simulink model "sampleModel1801"  (R2022a)
settings: Solver=FixedStepAuto  StartTime=0.0  StopTime=10.0  RelTol=1e-3
undefined symbols (not defined in the file): DiscIntNeverNeededParam, Newton, Raphson
libraries: simulink x66, slpidlib x17
(part 1 of 3)
settings Model: SimulationMode=software-in-the-loop (sil)  Creator=lenovo  LastModifiedBy=TSMC
settings DataIOCC: InspectSignalLogs=on  SignalLoggingName=logsOut
settings OptimizationCC: DefaultParameterBehavior=Inlined  EnhancedBackFolding=on  PassReuseOutputArgsAs=Individual arguments  ZeroExternalMemoryAtStartup=off  ZeroInternalMemoryAtStartup=off  OptimizeBlockOrder=speed  DifferentSizesBufferReuse=on  OptimizationCustomize=off  EfficientTunableParamExpr=on
settings DebuggingCC: ParameterTunabilityLossMsg=error  UnconnectedInputMsg=warning  UnconnectedOutputMsg=warning  UnconnectedLineMsg=warning
settings ModelReferenceCC: UpdateModelReferenceTargets=Force
settings SFSimCC: MATLABDynamicMemAlloc=off
settings RTWCC: SystemTargetFile=ert.tlc  TemplateMakefile=ert_default_tmf  GenerateReport=on  IncludeHyperlinkInReport=on  GenerateTraceInfo=on  DLArmComputeVersion=19.05
settings CodeAppCC: ForceParamTrailComments=on  IgnoreCustomStorageClasses=off  OperatorAnnotations=on  SimulinkDataObjDesc=on  SFDataObjDesc=on  InsertBlockDesc=on
settings ERTTargetCC: TargetLangStandard=C99 (ISO)  GenerateSampleERTMain=on  SupportContinuousTime=on  InlinedParameterPlacement=NonHierarchical  ERTCustomFileTemplate=example_file_process.tlc

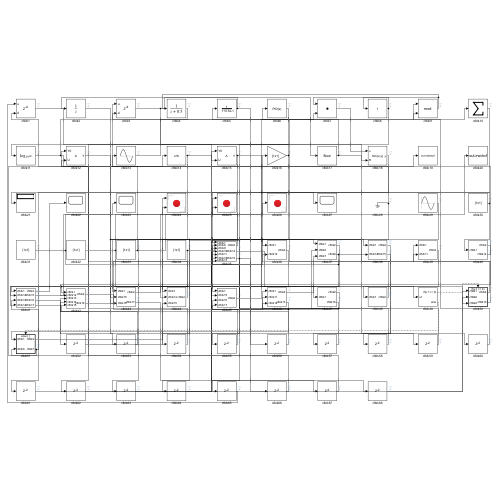
[thumbnail: Simulink's stored preview of the top-level diagram]
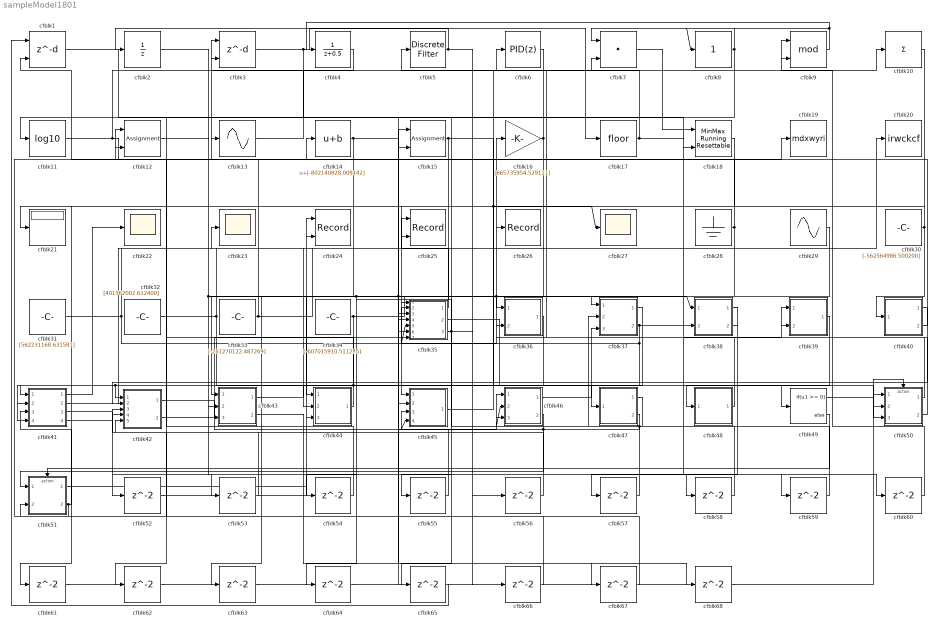
== system sampleModel1801 ==
  cfblk1 : Delay  DelayLengthSource=Input port  SampleTime=1
      settings: InputPortMap=u0,p1
  cfblk10 : Sum  Inputs=+
  cfblk11 : Math  Operator=log10
  cfblk12 : Assignment  DiagnosticForDimensions=Warning  IndexOptions=Index vector (dialog)  Indices=1  OutputSizes=1
  cfblk13 : Sin  TimeSource=Use external signal  SampleTime=0
  cfblk14 : Bias  Bias=[-802140828.008142]  SaturateOnIntegerOverflow=off
  cfblk15 : Assignment  DiagnosticForDimensions=Warning  IndexOptions=Index vector (dialog)  Indices=1  OutputSizes=1
  cfblk16 : Gain  Gain=[665735954.529111]
  cfblk17 : Rounding
  cfblk18 : simulink/Math Operations/MinMax Running Resettable  Function=min  vinit=0.0
  cfblk19 : ToWorkspace  VariableName=mdxwyri  SaveFormat=Timeseries  SampleTime=-1
  cfblk2 : UnitDelay  HasFrameUpgradeWarning=on
  cfblk20 : ToWorkspace  VariableName=irwckcf  SaveFormat=Timeseries  SampleTime=-1
  cfblk21 : Display
  cfblk22 : Scope
  cfblk23 : Scope
  cfblk24 : Record  FileSettingsInternal="{\"entries\":[{\"content\":{\"excelSettings\":{\"content\":{},\"type\":\"Streamout.ExcelSettings\"}},\"type\":\"Streamout.FileSettingStorage\",\"uuid\":\"da407134-930a-4060-90fa-d972cd5884a4\"}],\"packageUris\":[\"http://schema.mathworks.com/mf0/streamout_blocks/R2020a\"],\"version\":\"1.0\"}"  Layout=[1 1]  SignalsInternal="{\"entries\":[{\"content\":{\"signals\":[]},\"type\":\"RecordBlkView.InputSignals\",\"uuid\":\"b8d77bba-2430-47da-b420-9572af3fcd64\"}],\"packageUris\":[\"http://schema.mathworks.com/mf0/streamout_blocks/R2020a\"],\"version\":\"1.0\"}"  VisualizationBindings="{\"xyplotplugin\":{\"info\":[{\"series\":[],\"subplotID\":1}]}}"  CompatibilityTag=XY  st=-1
  cfblk25 : Record  FileSettingsInternal="{\"entries\":[{\"content\":{\"excelSettings\":{\"content\":{},\"type\":\"Streamout.ExcelSettings\"}},\"type\":\"Streamout.FileSettingStorage\",\"uuid\":\"0478fcfe-5d0e-44ee-9fcd-b61e8d59bef5\"}],\"packageUris\":[\"http://schema.mathworks.com/mf0/streamout_blocks/R2020a\"],\"version\":\"1.0\"}"  Layout=[1 1]  SignalsInternal="{\"entries\":[{\"content\":{\"signals\":[]},\"type\":\"RecordBlkView.InputSignals\",\"uuid\":\"ba91bab0-cdaa-4586-8070-7859b16663df\"}],\"packageUris\":[\"http://schema.mathworks.com/mf0/streamout_blocks/R2020a\"],\"version\":\"1.0\"}"  VisualizationBindings="{\"xyplotplugin\":{\"info\":[{\"series\":[],\"subplotID\":1}]}}"  CompatibilityTag=XY  st=-1
  cfblk26 : Record  FileSettingsInternal="{\"entries\":[{\"content\":{\"excelSettings\":{\"content\":{},\"type\":\"Streamout.ExcelSettings\"}},\"type\":\"Streamout.FileSettingStorage\",\"uuid\":\"70eb35dc-156c-423f-ab29-1b62ce158527\"}],\"packageUris\":[\"http://schema.mathworks.com/mf0/streamout_blocks/R2020a\"],\"version\":\"1.0\"}"  SignalsInternal="{\"entries\":[{\"content\":{\"signals\":[]},\"type\":\"RecordBlkView.InputSignals\",\"uuid\":\"3f0c1e90-9f95-4c65-babb-aeb54cbaeaf7\"}],\"packageUris\":[\"http://schema.mathworks.com/mf0/streamout_blocks/R2020a\"],\"version\":\"1.0\"}"  VisualizationBindings="{\"sparklinesplugin\":{\"info\":[{\"bindingParametersList\":[],\"subplotID\":1}]}}"
  cfblk27 : Scope
  cfblk28 : Ground
  cfblk29 : Sin  Amplitude=[684888808.035051]  Bias=[-873630201.820867]  SampleTime=0
  cfblk3 : Delay  DelayLengthSource=Input port  SampleTime=1
      settings: InputPortMap=u0,p1
  cfblk30 : Constant  Value=[-562564986.500200]  SampleTime=1
  cfblk31 : Constant  Value=[562231168.631581]  SampleTime=1
  cfblk32 : Constant  Value=[401562002.612400]  SampleTime=1
  cfblk33 : Constant  Value=[-251270122.487269]  SampleTime=1
  cfblk34 : Constant  Value=[-607015910.511275]  SampleTime=1
  cfblk35 : Subsystem
  cfblk36 : Subsystem
  cfblk37 : Subsystem
  cfblk38 : Subsystem
  cfblk39 : Subsystem
  cfblk4 : DiscreteTransferFcn  SampleTime=1
  cfblk40 : Subsystem
  cfblk41 : Subsystem
  cfblk42 : Subsystem
  cfblk43 : Subsystem
  cfblk44 : Subsystem
  cfblk45 : Subsystem
  cfblk46 : Subsystem
  cfblk47 : Subsystem
  cfblk48 : Subsystem
  cfblk49 : If  IfExpression=u1 >= 0  SampleTime=1
  cfblk5 : DiscreteFilter  SampleTime=1
  cfblk50 : Subsystem  TreatAsAtomicUnit=on
  cfblk51 : Subsystem  TreatAsAtomicUnit=on
  cfblk{52..68} (17 alike) : Delay  SampleTime=1
  cfblk6 : slpidlib/PID Controller  Controller=PID  Form=Parallel  TimeDomain=Discrete-time  UseExternalTs=off  SampleTime=1  IntegratorMethod=Forward Euler  FilterMethod=Forward Euler  ControllerParametersSource=internal  P=1  I=1  UseKiTs=off  D=0  N=100  UseFilter=on  TunerSelectOption=Transfer Function Based (PID Tuner App)  InitialConditionSource=internal  InitialConditionForIntegrator=0  InitialConditionForFilter=0  DifferentiatorICPrevScaledInput=0  ExternalReset=none  TrackingMode=off  Kt=1  LimitOutput=off  SatLimitsSource=internal  UpperSaturationLimit=inf  LowerSaturationLimit=-inf  LinearizeAsGain=off  AntiWindupMode=none  Kb=1  POutMin=[]  POutMax=[]  IOutMin=[]  IOutMax=[]  DOutMin=[]  DOutMax=[]  NOutMin=[]  NOutMax=[]  SumOutMin=[]  SumOutMax=[]  SaturationOutMin=[]  SaturationOutMax=[]  PParamMin=[]  PParamMax=[]  IParamMin=[]  IParamMax=[]  DParamMin=[]  DParamMax=[]  NParamMin=[]  NParamMax=[]  KbParamMin=[]  KbParamMax=[]  KtParamMin=[]  KtParamMax=[]  KbOutMin=[]  KbOutMax=[]  KtOutMin=[]  KtOutMax=[]  IntegratorOutMin=[]  IntegratorOutMax=[]  FilterOutMin=[]  FilterOutMax=[]  SumI1OutMin=[]  SumI1OutMax=[]  SumI2OutMin=[]  SumI2OutMax=[]  SumI3OutMin=[]  SumI3OutMax=[]  SumI4OutMin=[]  SumI4OutMax=[]  SumDOutMin=[]  SumDOutMax=[]  DifferentiatorOutMin=[]  DifferentiatorOutMax=[]  FilterDiffOutCoefMin=[]  FilterDiffOutCoefMax=[]  ReciprocalOutMin=[]  ReciprocalOutMax=[]  SumDenOutMin=[]  SumDenOutMax=[]  SumNumOutMin=[]  SumNumOutMax=[]  DivideOutMin=[]  DivideOutMax=[]  UdiffTsProdOutMin=[]  UdiffTsProdOutMax=[]  NTsProdOutMin=[]  NTsProdOutMax=[]  UintegralTsProdOutMin=[]  UintegralTsProdOutMax=[]  UngainTsProdOutMin=[]  UngainTsProdOutMax=[]  IntegratorContinuousStateAttributes=''  IntegratorStateMustResolveToSignalObject=off  IntegratorRTWStateStorageClass=Auto  FilterContinuousStateAttributes=''  FilterStateMustResolveToSignalObject=off  FilterRTWStateStorageClass=Auto  ParallelPVariant=InternalParameters  IdealPVariant=Disabled  IVariant=InternalParameters  DVariant=InternalParameters  IntegratorVariant=Discrete  SatVariant=Disabled  AWVariant=Passthrough  PCopyVariant=Disabled  TRVariant=Disabled  FdbkBlocksVariant=Forward  IdealPFdbkVariant=Disabled  SatFdbkVariant=Disabled  DerivativeFilterVariant=ForwardEulerFilter  NVariant=InternalParameters  NCopyVariant=Disabled  FilterICVariant=InternalICsFilter  IntegratorICVariant=InternalICs  ExternalResetVariant=Disabled  TRSumVariant=Passthrough  SumFdbkVariant=Disabled  SumVariant=Sum_PID  TsampFilterVariant=InternalTs  TsampNgainVariant=Passthrough  TsampIntegralVariant=Passthrough  ExternalSaturationOutDataTypeStr=Inherit: Same as second input  aMode=0
  cfblk7 : DotProduct  OutDataTypeStr=Inherit: Inherit via internal rule
  cfblk8 : simulink/Math Operations/Slider Gain  gain=1  low=0  high=2
  cfblk9 : Math  Operator=mod
  wires:
  cfblk10/1 -> cfblk45/1(cfblk1)
  cfblk51/1(cfblk2) -> cfblk24/1
  cfblk34/1 -> cfblk37/1(cfblk1), cfblk43/2(cfblk15)
  cfblk8/1 -> cfblk7/1, cfblk62/1
  cfblk29/1 -> cfblk44/1(cfblk1)
  cfblk46/1(cfblk2) -> cfblk37/3(cfblk7)
  cfblk3/1 -> cfblk17/1, cfblk18/2
  cfblk41/1(cfblk2) -> cfblk22/1
  cfblk30/1 -> cfblk21/1, cfblk40/1(cfblk1)
  cfblk50/1(cfblk2) -> cfblk16/1
  cfblk41/2(cfblk15) -> cfblk20/1
  cfblk7/1 -> cfblk18/1
  cfblk47/1(cfblk2) -> cfblk46/1(cfblk1)
  cfblk39/1(cfblk2) -> cfblk48/1(cfblk1)
  cfblk4/1 -> cfblk3/1
  cfblk32/1 -> cfblk24/2, cfblk49/1
  cfblk50/2(cfblk10) -> cfblk39/1(cfblk1)
  cfblk47/2(cfblk16) -> cfblk46/2(cfblk11), cfblk45/3(cfblk16)
  cfblk15/1 -> cfblk27/1, cfblk47/1(cfblk1), cfblk44/2(cfblk14)
  cfblk51/2(cfblk7) -> cfblk14/1, cfblk41/3(cfblk13)
  cfblk44/1(cfblk2) -> cfblk12/1, cfblk41/2(cfblk12)
  cfblk36/1(cfblk2) -> cfblk42/1(cfblk1), cfblk41/4(cfblk14)
  cfblk28/1 -> cfblk3/2, cfblk43/3(cfblk16)
  cfblk1/1 -> cfblk15/2
  cfblk46/2(cfblk13) -> cfblk51/1(cfblk1), cfblk45/4(cfblk17)
  cfblk17/1 -> cfblk5/1, cfblk60/1
  cfblk37/1(cfblk2) -> cfblk41/1(cfblk1)
  cfblk48/1(cfblk2) -> cfblk6/1
  cfblk11/1 -> cfblk19/1, cfblk9/1
  cfblk45/1(cfblk2) -> cfblk7/2
  cfblk33/1 -> cfblk25/1, cfblk1/2
  cfblk2/1 -> cfblk38/1(cfblk1), cfblk59/1
  cfblk42/1(cfblk2) -> cfblk46/3(cfblk12)
  cfblk40/1(cfblk2) -> cfblk42/2(cfblk12)
  cfblk16/1 -> cfblk63/1, cfblk64/1, cfblk45/2(cfblk15), cfblk11/1
  cfblk43/1(cfblk2) -> cfblk26/1
  cfblk37/2(cfblk8) -> cfblk35/5(cfblk11), cfblk54/1, cfblk39/2(cfblk11)
  cfblk9/1 -> cfblk4/1, cfblk8/1
  cfblk13/1 -> cfblk10/1
  cfblk14/1 -> cfblk43/1(cfblk1), cfblk67/1
  cfblk40/2(cfblk12) -> cfblk13/1
  cfblk5/1 -> cfblk2/1, cfblk56/1
  cfblk42/2(cfblk16) -> cfblk35/2(cfblk8)
  cfblk35/1(cfblk2) -> cfblk25/2
  cfblk12/1 -> cfblk36/1(cfblk1), cfblk38/2(cfblk14)
  cfblk35/2(cfblk14) -> cfblk50/3(cfblk9)
  cfblk31/1 -> cfblk36/2(cfblk14), cfblk23/1
  cfblk35/3(cfblk15) -> cfblk65/1, cfblk66/1
  cfblk49/1 -> cfblk50/Action
  cfblk49/2 -> cfblk51/Action
  cfblk41/3(cfblk16) -> cfblk52/1
  cfblk52/1 -> cfblk44/3(cfblk15)
  cfblk41/4(cfblk17) -> cfblk53/1
  cfblk53/1 -> cfblk42/4(cfblk14)
  cfblk54/1 -> cfblk12/2
  cfblk6/1 -> cfblk55/1
  cfblk55/1 -> cfblk15/1
  cfblk56/1 -> cfblk42/3(cfblk13)
  cfblk38/1(cfblk2) -> cfblk57/1
  cfblk57/1 -> cfblk37/2(cfblk6)
  cfblk38/2(cfblk15) -> cfblk58/1
  cfblk58/1 -> cfblk35/1(cfblk1)
  cfblk59/1 -> cfblk35/7(cfblk13)
  cfblk60/1 -> cfblk9/2
  cfblk18/1 -> cfblk61/1
  cfblk61/1 -> cfblk50/1(cfblk1)
  cfblk62/1 -> cfblk35/4(cfblk10)
  cfblk63/1 -> cfblk35/3(cfblk9)
  cfblk64/1 -> cfblk35/6(cfblk12)
  cfblk65/1 -> cfblk1/1
  cfblk66/1 -> cfblk42/5(cfblk15)
  cfblk67/1 -> cfblk51/2(cfblk6)
  cfblk43/2(cfblk17) -> cfblk68/1
  cfblk68/1 -> cfblk50/2(cfblk8)

== system sampleModel1801/cfblk35 ==
  cfblk1 : Inport
  cfblk8 : Inport  Port=2
  cfblk9 : Inport  Port=3
  cfblk10 : Inport  Port=4
  cfblk11 : Inport  Port=5
  cfblk12 : Inport  Port=6
  cfblk13 : Inport  Port=7
  cfblk3 : DiscreteZeroPole  Poles=[0 0.5]  Gain=1
  cfblk4 : Sum  Inputs=+
  cfblk5 : PermuteDimensions
  cfblk6 : Constant  Value=[-592343644.512658]  SampleTime=1
  cfblk7 : Subsystem
  cfblk2 : Outport
  cfblk14 : Outport  Port=2
  cfblk15 : Outport  Port=3
  wires:
  cfblk5/1 -> cfblk15/1
  cfblk9/1 -> cfblk4/1
  cfblk13/1 -> cfblk14/1
  cfblk12/1 -> cfblk7/1(cfblk1)
  cfblk3/1 -> cfblk7/2(cfblk13)
  cfblk6/1 -> cfblk5/1
  cfblk11/1 -> cfblk7/3(cfblk14)
  cfblk4/1 -> cfblk2/1
  cfblk8/1 -> cfblk3/1

== system sampleModel1801/cfblk36 ==
  cfblk1 : Inport
  cfblk14 : Inport  Port=2
  cfblk10 : Subsystem
  cfblk11 : Subsystem
  cfblk12 : Subsystem
  cfblk13 : Subsystem
  cfblk15 : Delay  SampleTime=1
  cfblk16 : Delay  SampleTime=1
  cfblk3 : DiscreteFir  SampleTime=1
  cfblk4 : ComplexToRealImag
  cfblk5 : ComplexToRealImag
  cfblk6 : Abs  SaturateOnIntegerOverflow=off
  cfblk7 : Bias  Bias=[-287900878.925501]  SaturateOnIntegerOverflow=off
  cfblk8 : ComplexToMagnitudeAngle
  cfblk9 : Constant  Value=[628563794.739132]  SampleTime=1
  cfblk2 : Outport
  wires:
  cfblk12/1(cfblk2) -> cfblk8/1
  cfblk6/1 -> cfblk12/1(cfblk1)
  cfblk5/1 -> cfblk7/1
  cfblk7/1 -> cfblk2/1, cfblk13/2(cfblk8)
  cfblk14/1 -> cfblk5/1
  cfblk8/1 -> cfblk3/1
  cfblk9/1 -> cfblk10/1(cfblk1)
  cfblk1/1 -> cfblk11/2(cfblk13)
  cfblk11/1(cfblk2) -> cfblk6/1
  cfblk10/1(cfblk2) -> cfblk12/2(cfblk11)
  cfblk11/2(cfblk16) -> cfblk10/2(cfblk11)
  cfblk5/2 -> cfblk12/3(cfblk12), cfblk4/1
  cfblk11/3(cfblk17) -> cfblk10/3(cfblk12)
  cfblk4/1 -> cfblk12/4(cfblk13)
  cfblk4/2 -> cfblk13/1(cfblk1)
  cfblk13/1(cfblk2) -> cfblk12/5(cfblk14)
  cfblk13/2(cfblk9) -> cfblk12/6(cfblk15)
  cfblk13/3(cfblk10) -> cfblk11/4(cfblk15)
  cfblk3/1 -> cfblk15/1
  cfblk15/1 -> cfblk11/1(cfblk1)
  cfblk8/2 -> cfblk16/1
  cfblk16/1 -> cfblk11/3(cfblk14)

== system sampleModel1801/cfblk37 ==
  cfblk1 : Inport
  cfblk6 : Inport  Port=2
  cfblk7 : Inport  Port=3
  cfblk3 : DiscreteFilter  SampleTime=1
  cfblk4 : ComplexToMagnitudeAngle
  cfblk5 : Squeeze
  cfblk9 : Delay  SampleTime=1
  cfblk2 : Outport
  cfblk8 : Outport  Port=2
  wires:
  cfblk1/1 -> cfblk8/1
  cfblk3/1 -> cfblk4/1
  cfblk4/1 -> cfblk5/1
  cfblk4/2 -> cfblk2/1
  cfblk5/1 -> cfblk9/1
  cfblk9/1 -> cfblk3/1

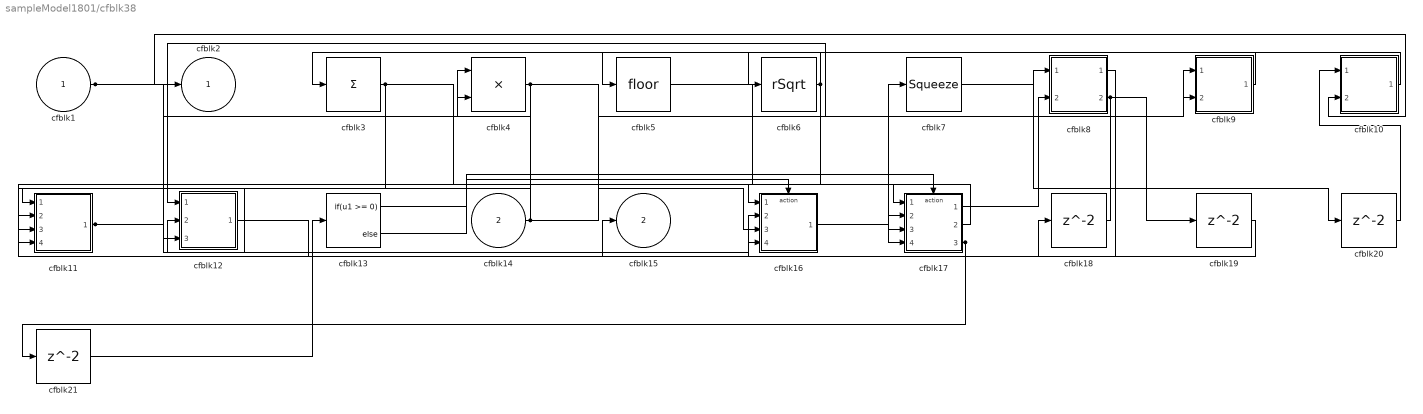
== system sampleModel1801/cfblk38 ==
  cfblk1 : Inport
  cfblk14 : Inport  Port=2
  cfblk10 : Subsystem
  cfblk11 : Subsystem
  cfblk12 : Subsystem
  cfblk13 : If  IfExpression=u1 >= 0  SampleTime=1
  cfblk16 : Subsystem  TreatAsAtomicUnit=on
  cfblk17 : Subsystem  TreatAsAtomicUnit=on
  cfblk{18..21} (4 alike) : Delay  SampleTime=1
  cfblk3 : Sum  Inputs=+
  cfblk4 : Product  Inputs=**
  cfblk5 : Rounding
  cfblk6 : Sqrt  Operator=rSqrt  AlgorithmType=Newton-Raphson
  cfblk7 : Squeeze
  cfblk8 : Subsystem
  cfblk9 : Subsystem
  cfblk2 : Outport
  cfblk15 : Outport  Port=2
  wires:
  cfblk5/1 -> cfblk17/1(cfblk1)
  cfblk6/1 -> cfblk3/1, cfblk11/4(cfblk16)
  cfblk8/1(cfblk2) -> cfblk15/1
  cfblk8/2(cfblk7) -> cfblk12/1(cfblk1), cfblk19/1
  cfblk4/1 -> cfblk12/2(cfblk13), cfblk16/3(cfblk11), cfblk17/4(cfblk12)
  cfblk14/1 -> cfblk4/1, cfblk9/1(cfblk1), cfblk9/2(cfblk15)
  cfblk3/1 -> cfblk11/1(cfblk1), cfblk12/3(cfblk14), cfblk17/3(cfblk11), cfblk11/3(cfblk15)
  cfblk10/1(cfblk2) -> cfblk6/1
  cfblk17/1(cfblk2) -> cfblk8/2(cfblk6)
  cfblk11/1(cfblk2) -> cfblk2/1, cfblk17/2(cfblk10), cfblk16/4(cfblk12)
  cfblk16/1(cfblk2) -> cfblk7/1
  cfblk1/1 -> cfblk10/2(cfblk11), cfblk4/2
  cfblk9/1(cfblk2) -> cfblk5/1
  cfblk17/2(cfblk13) -> cfblk16/1(cfblk1)
  cfblk17/3(cfblk14) -> cfblk16/2(cfblk10), cfblk21/1
  cfblk13/1 -> cfblk16/Action
  cfblk13/2 -> cfblk17/Action
  cfblk12/1(cfblk2) -> cfblk18/1
  cfblk18/1 -> cfblk8/1(cfblk1)
  cfblk19/1 -> cfblk11/2(cfblk14)
  cfblk7/1 -> cfblk20/1
  cfblk20/1 -> cfblk10/1(cfblk1)
  cfblk21/1 -> cfblk13/1

== system sampleModel1801/cfblk39 ==
  cfblk1 : Inport
  cfblk11 : Inport  Port=2
  cfblk10 : Subsystem
  cfblk12 : Delay  SampleTime=1
  cfblk3 : slpidlib/PID Controller  Controller=PID  Form=Parallel  TimeDomain=Discrete-time  UseExternalTs=off  SampleTime=1  IntegratorMethod=Forward Euler  FilterMethod=Forward Euler  ControllerParametersSource=internal  P=1  I=1  UseKiTs=off  D=0  N=100  UseFilter=on  TunerSelectOption=Transfer Function Based (PID Tuner App)  InitialConditionSource=internal  InitialConditionForIntegrator=0  InitialConditionForFilter=0  DifferentiatorICPrevScaledInput=0  ExternalReset=none  TrackingMode=off  Kt=1  LimitOutput=off  SatLimitsSource=internal  UpperSaturationLimit=inf  LowerSaturationLimit=-inf  LinearizeAsGain=off  AntiWindupMode=none  Kb=1  POutMin=[]  POutMax=[]  IOutMin=[]  IOutMax=[]  DOutMin=[]  DOutMax=[]  NOutMin=[]  NOutMax=[]  SumOutMin=[]  SumOutMax=[]  SaturationOutMin=[]  SaturationOutMax=[]  PParamMin=[]  PParamMax=[]  IParamMin=[]  IParamMax=[]  DParamMin=[]  DParamMax=[]  NParamMin=[]  NParamMax=[]  KbParamMin=[]  KbParamMax=[]  KtParamMin=[]  KtParamMax=[]  KbOutMin=[]  KbOutMax=[]  KtOutMin=[]  KtOutMax=[]  IntegratorOutMin=[]  IntegratorOutMax=[]  FilterOutMin=[]  FilterOutMax=[]  SumI1OutMin=[]  SumI1OutMax=[]  SumI2OutMin=[]  SumI2OutMax=[]  SumI3OutMin=[]  SumI3OutMax=[]  SumI4OutMin=[]  SumI4OutMax=[]  SumDOutMin=[]  SumDOutMax=[]  DifferentiatorOutMin=[]  DifferentiatorOutMax=[]  FilterDiffOutCoefMin=[]  FilterDiffOutCoefMax=[]  ReciprocalOutMin=[]  ReciprocalOutMax=[]  SumDenOutMin=[]  SumDenOutMax=[]  SumNumOutMin=[]  SumNumOutMax=[]  DivideOutMin=[]  DivideOutMax=[]  UdiffTsProdOutMin=[]  UdiffTsProdOutMax=[]  NTsProdOutMin=[]  NTsProdOutMax=[]  UintegralTsProdOutMin=[]  UintegralTsProdOutMax=[]  UngainTsProdOutMin=[]  UngainTsProdOutMax=[]  IntegratorContinuousStateAttributes=''  IntegratorStateMustResolveToSignalObject=off  IntegratorRTWStateStorageClass=Auto  FilterContinuousStateAttributes=''  FilterStateMustResolveToSignalObject=off  FilterRTWStateStorageClass=Auto  ParallelPVariant=InternalParameters  IdealPVariant=Disabled  IVariant=InternalParameters  DVariant=InternalParameters  IntegratorVariant=Discrete  SatVariant=Disabled  AWVariant=Passthrough  PCopyVariant=Disabled  TRVariant=Disabled  FdbkBlocksVariant=Forward  IdealPFdbkVariant=Disabled  SatFdbkVariant=Disabled  DerivativeFilterVariant=ForwardEulerFilter  NVariant=InternalParameters  NCopyVariant=Disabled  FilterICVariant=InternalICsFilter  IntegratorICVariant=InternalICs  ExternalResetVariant=Disabled  TRSumVariant=Passthrough  SumFdbkVariant=Disabled  SumVariant=Sum_PID  TsampFilterVariant=InternalTs  TsampNgainVariant=Passthrough  TsampIntegralVariant=Passthrough  ExternalSaturationOutDataTypeStr=Inherit: Same as second input  aMode=0
  cfblk4 : Sum  Inputs=+
  cfblk5 : Sum  Inputs=+-
  cfblk6 : Bias  Bias=[231218771.259830]  SaturateOnIntegerOverflow=off
  cfblk7 : Squeeze
  cfblk8 : Subsystem
  cfblk9 : Subsystem
  cfblk2 : Outport
  wires:
  cfblk1/1 -> cfblk4/1
  cfblk6/1 -> cfblk9/1(cfblk1)
  cfblk8/1(cfblk2) -> cfblk3/1
  cfblk3/1 -> cfblk2/1
  cfblk11/1 -> cfblk8/1(cfblk1)
  cfblk10/1(cfblk2) -> cfblk6/1
  cfblk7/1 -> cfblk5/1, cfblk10/1(cfblk1)
  cfblk4/1 -> cfblk8/2(cfblk8)
  cfblk10/2(cfblk11) -> cfblk9/2(cfblk16)
  cfblk9/1(cfblk2) -> cfblk5/2
  cfblk10/4(cfblk13) -> cfblk9/3(cfblk17)
  cfblk5/1 -> cfblk8/3(cfblk9), cfblk8/4(cfblk10)
  cfblk10/3(cfblk12) -> cfblk12/1
  cfblk12/1 -> cfblk7/1

== system sampleModel1801/cfblk40 ==
  cfblk1 : Inport
  cfblk10 : Subsystem
  cfblk11 : Subsystem
  cfblk13 : Delay  SampleTime=1
  cfblk14 : Delay  SampleTime=1
  cfblk3 : DiscreteTransferFcn  SampleTime=1
  cfblk4 : DiscreteFir  SampleTime=1
  cfblk5 : Sum  Inputs=+
  cfblk6 : Assignment  DiagnosticForDimensions=Warning  IndexOptions=Index vector (dialog)  Indices=1  OutputSizes=1
  cfblk7 : Constant  Value=[-706275241.010512]  SampleTime=1
  cfblk8 : Constant  Value=[815598875.287357]  SampleTime=1
  cfblk9 : Constant  Value=[-123317934.757215]  SampleTime=1
  cfblk2 : Outport
  cfblk12 : Outport  Port=2
  wires:
  cfblk10/1(cfblk2) -> cfblk3/1
  cfblk9/1 -> cfblk11/1(cfblk1)
  cfblk11/1(cfblk2) -> cfblk2/1
  cfblk1/1 -> cfblk11/2(cfblk11)
  cfblk6/1 -> cfblk12/1, cfblk5/1
  cfblk8/1 -> cfblk11/3(cfblk12)
  cfblk11/2(cfblk13) -> cfblk6/1, cfblk10/4(cfblk13)
  cfblk7/1 -> cfblk10/2(cfblk11)
  cfblk4/1 -> cfblk10/3(cfblk12)
  cfblk5/1 -> cfblk4/1, cfblk14/1
  cfblk3/1 -> cfblk13/1
  cfblk13/1 -> cfblk10/1(cfblk1)
  cfblk14/1 -> cfblk6/2

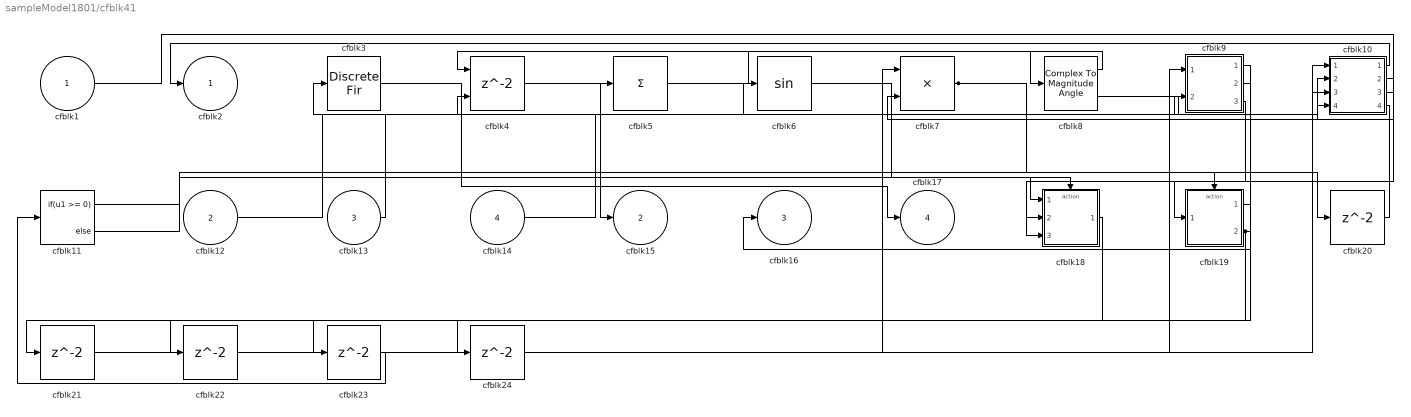
== system sampleModel1801/cfblk41 ==
  cfblk1 : Inport
  cfblk12 : Inport  Port=2
  cfblk13 : Inport  Port=3
  cfblk14 : Inport  Port=4
  cfblk10 : Subsystem
  cfblk11 : If  IfExpression=u1 >= 0  SampleTime=1
  cfblk18 : Subsystem  TreatAsAtomicUnit=on
  cfblk19 : Subsystem  TreatAsAtomicUnit=on
  cfblk{20..24} (5 alike) : Delay  SampleTime=1
  cfblk3 : DiscreteFir  SampleTime=1
  cfblk4 : Delay  ShowEnablePort=on  SampleTime=1
      settings: InputPortMap=u0,e6
  cfblk5 : Sum  Inputs=+
  cfblk6 : Trigonometry
  cfblk7 : Product  Inputs=**
  cfblk8 : ComplexToMagnitudeAngle
  cfblk9 : Subsystem
  cfblk2 : Outport
  cfblk15 : Outport  Port=2
  cfblk16 : Outport  Port=3
  cfblk17 : Outport  Port=4
  wires:
  cfblk3/1 -> cfblk17/1
  cfblk13/1 -> cfblk3/1
  cfblk6/1 -> cfblk18/1(cfblk1)
  cfblk4/1 -> cfblk15/1
  cfblk12/1 -> cfblk5/1
  cfblk5/1 -> cfblk8/1
  cfblk10/1(cfblk2) -> cfblk2/1
  cfblk9/1(cfblk2) -> cfblk16/1
  cfblk7/1 -> cfblk9/2(cfblk8), cfblk20/1
  cfblk14/1 -> cfblk6/1
  cfblk9/3(cfblk10) -> cfblk19/1(cfblk1)
  cfblk1/1 -> cfblk10/2(cfblk12)
  cfblk10/2(cfblk15) -> cfblk7/2
  cfblk8/1 -> cfblk4/1
  cfblk8/2 -> cfblk10/4(cfblk14)
  cfblk19/2(cfblk9) -> cfblk4/2, cfblk24/1
  cfblk10/3(cfblk16) -> cfblk18/2(cfblk9)
  cfblk10/4(cfblk17) -> cfblk18/3(cfblk10)
  cfblk11/1 -> cfblk18/Action
  cfblk11/2 -> cfblk19/Action
  cfblk20/1 -> cfblk10/1(cfblk1)
  cfblk9/2(cfblk9) -> cfblk21/1
  cfblk21/1 -> cfblk7/1
  cfblk18/1(cfblk2) -> cfblk22/1
  cfblk22/1 -> cfblk10/3(cfblk13)
  cfblk19/1(cfblk2) -> cfblk23/1
  cfblk23/1 -> cfblk11/1
  cfblk24/1 -> cfblk9/1(cfblk1)

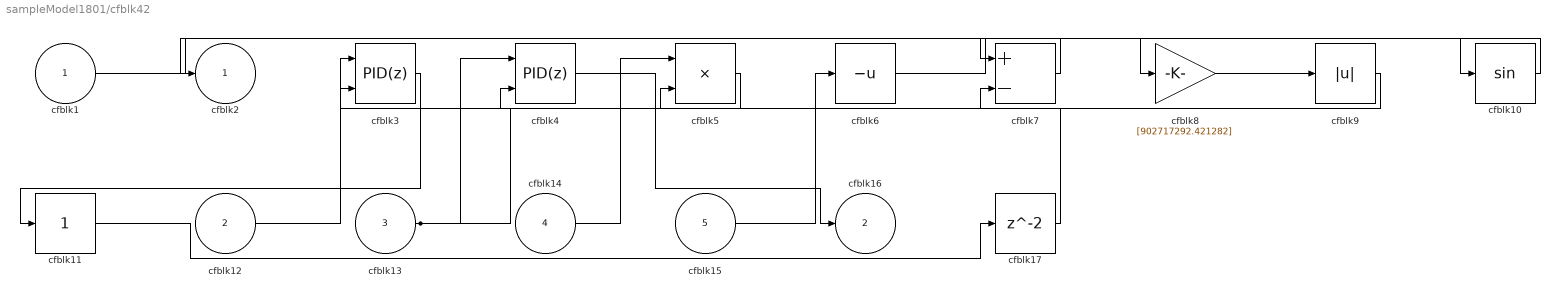
== system sampleModel1801/cfblk42 ==
  cfblk1 : Inport
  cfblk12 : Inport  Port=2
  cfblk13 : Inport  Port=3
  cfblk14 : Inport  Port=4
  cfblk15 : Inport  Port=5
  cfblk10 : Trigonometry
  cfblk11 : simulink/Math Operations/Slider Gain  gain=1  low=0  high=2
  cfblk17 : Delay  SampleTime=1
  cfblk3 : slpidlib/PID Controller (2DOF)  Controller=PID  Form=Parallel  TimeDomain=Discrete-time  UseExternalTs=off  SampleTime=1  IntegratorMethod=Forward Euler  FilterMethod=Forward Euler  ControllerParametersSource=internal  P=1  I=1  UseKiTs=off  D=0  N=100  UseFilter=on  b=1  c=1  TunerSelectOption=Transfer Function Based (PID Tuner App)  InitialConditionSource=internal  InitialConditionForIntegrator=0  InitialConditionForFilter=0  DifferentiatorICPrevScaledInput=0  ExternalReset=none  TrackingMode=off  Kt=1  LimitOutput=off  SatLimitsSource=internal  UpperSaturationLimit=inf  LowerSaturationLimit=-inf  LinearizeAsGain=off  AntiWindupMode=none  Kb=1  POutMin=[]  POutMax=[]  IOutMin=[]  IOutMax=[]  DOutMin=[]  DOutMax=[]  NOutMin=[]  NOutMax=[]  bOutMin=[]  bOutMax=[]  cOutMin=[]  cOutMax=[]  SumOutMin=[]  SumOutMax=[]  SaturationOutMin=[]  SaturationOutMax=[]  PParamMin=[]  PParamMax=[]  IParamMin=[]  IParamMax=[]  DParamMin=[]  DParamMax=[]  NParamMin=[]  NParamMax=[]  bParamMin=[]  bParamMax=[]  cParamMin=[]  cParamMax=[]  KbParamMin=[]  KbParamMax=[]  KtParamMin=[]  KtParamMax=[]  KbOutMin=[]  KbOutMax=[]  KtOutMin=[]  KtOutMax=[]  IntegratorOutMin=[]  IntegratorOutMax=[]  FilterOutMin=[]  FilterOutMax=[]  SumI1OutMin=[]  SumI1OutMax=[]  SumI2OutMin=[]  SumI2OutMax=[]  SumI3OutMin=[]  SumI3OutMax=[]  SumI4OutMin=[]  SumI4OutMax=[]  SumDOutMin=[]  SumDOutMax=[]  Sum1OutMin=[]  Sum1OutMax=[]  Sum2OutMin=[]  Sum2OutMax=[]  Sum3OutMin=[]  Sum3OutMax=[]  DifferentiatorOutMin=[]  DifferentiatorOutMax=[]  FilterDiffOutCoefMin=[]  FilterDiffOutCoefMax=[]  ReciprocalOutMin=[]  ReciprocalOutMax=[]  SumDenOutMin=[]  SumDenOutMax=[]  SumNumOutMin=[]  SumNumOutMax=[]  DivideOutMin=[]  DivideOutMax=[]  UdiffTsProdOutMin=[]  UdiffTsProdOutMax=[]  NTsProdOutMin=[]  NTsProdOutMax=[]  UintegralTsProdOutMin=[]  UintegralTsProdOutMax=[]  UngainTsProdOutMin=[]  UngainTsProdOutMax=[]  IntegratorContinuousStateAttributes=''  IntegratorStateMustResolveToSignalObject=off  IntegratorRTWStateStorageClass=Auto  FilterContinuousStateAttributes=''  FilterStateMustResolveToSignalObject=off  FilterRTWStateStorageClass=Auto  ParallelPVariant=InternalParameters  IdealPVariant=Disabled  IVariant=InternalParameters  DVariant=InternalParameters  bVariant=InternalParameters  cVariant=InternalParameters  IntegratorVariant=Discrete  SatVariant=Disabled  AWVariant=Passthrough  PCopyVariant=Disabled  TRVariant=Disabled  FdbkBlocksVariant=Forward  IdealPFdbkVariant=Disabled  SatFdbkVariant=Disabled  DerivativeFilterVariant=ForwardEulerFilter  NVariant=InternalParameters  NCopyVariant=Disabled  FilterICVariant=InternalICsFilter  IntegratorICVariant=InternalICs  ExternalResetVariant=Disabled  TRSumVariant=Passthrough  SumFdbkVariant=Disabled  SumVariant=Sum_PID  TsampFilterVariant=InternalTs  TsampNgainVariant=Passthrough  TsampIntegralVariant=Passthrough  ExternalSaturationOutDataTypeStr=Inherit: Same as second input
      settings: SourceProductBaseCode=SL
  cfblk4 : slpidlib/PID Controller (2DOF)  Controller=PID  Form=Parallel  TimeDomain=Discrete-time  UseExternalTs=off  SampleTime=1  IntegratorMethod=Forward Euler  FilterMethod=Forward Euler  ControllerParametersSource=internal  P=1  I=1  UseKiTs=off  D=0  N=100  UseFilter=on  b=1  c=1  TunerSelectOption=Transfer Function Based (PID Tuner App)  InitialConditionSource=internal  InitialConditionForIntegrator=0  InitialConditionForFilter=0  DifferentiatorICPrevScaledInput=0  ExternalReset=none  TrackingMode=off  Kt=1  LimitOutput=off  SatLimitsSource=internal  UpperSaturationLimit=inf  LowerSaturationLimit=-inf  LinearizeAsGain=off  AntiWindupMode=none  Kb=1  POutMin=[]  POutMax=[]  IOutMin=[]  IOutMax=[]  DOutMin=[]  DOutMax=[]  NOutMin=[]  NOutMax=[]  bOutMin=[]  bOutMax=[]  cOutMin=[]  cOutMax=[]  SumOutMin=[]  SumOutMax=[]  SaturationOutMin=[]  SaturationOutMax=[]  PParamMin=[]  PParamMax=[]  IParamMin=[]  IParamMax=[]  DParamMin=[]  DParamMax=[]  NParamMin=[]  NParamMax=[]  bParamMin=[]  bParamMax=[]  cParamMin=[]  cParamMax=[]  KbParamMin=[]  KbParamMax=[]  KtParamMin=[]  KtParamMax=[]  KbOutMin=[]  KbOutMax=[]  KtOutMin=[]  KtOutMax=[]  IntegratorOutMin=[]  IntegratorOutMax=[]  FilterOutMin=[]  FilterOutMax=[]  SumI1OutMin=[]  SumI1OutMax=[]  SumI2OutMin=[]  SumI2OutMax=[]  SumI3OutMin=[]  SumI3OutMax=[]  SumI4OutMin=[]  SumI4OutMax=[]  SumDOutMin=[]  SumDOutMax=[]  Sum1OutMin=[]  Sum1OutMax=[]  Sum2OutMin=[]  Sum2OutMax=[]  Sum3OutMin=[]  Sum3OutMax=[]  DifferentiatorOutMin=[]  DifferentiatorOutMax=[]  FilterDiffOutCoefMin=[]  FilterDiffOutCoefMax=[]  ReciprocalOutMin=[]  ReciprocalOutMax=[]  SumDenOutMin=[]  SumDenOutMax=[]  SumNumOutMin=[]  SumNumOutMax=[]  DivideOutMin=[]  DivideOutMax=[]  UdiffTsProdOutMin=[]  UdiffTsProdOutMax=[]  NTsProdOutMin=[]  NTsProdOutMax=[]  UintegralTsProdOutMin=[]  UintegralTsProdOutMax=[]  UngainTsProdOutMin=[]  UngainTsProdOutMax=[]  IntegratorContinuousStateAttributes=''  IntegratorStateMustResolveToSignalObject=off  IntegratorRTWStateStorageClass=Auto  FilterContinuousStateAttributes=''  FilterStateMustResolveToSignalObject=off  FilterRTWStateStorageClass=Auto  ParallelPVariant=InternalParameters  IdealPVariant=Disabled  IVariant=InternalParameters  DVariant=InternalParameters  bVariant=InternalParameters  cVariant=InternalParameters  IntegratorVariant=Discrete  SatVariant=Disabled  AWVariant=Passthrough  PCopyVariant=Disabled  TRVariant=Disabled  FdbkBlocksVariant=Forward  IdealPFdbkVariant=Disabled  SatFdbkVariant=Disabled  DerivativeFilterVariant=ForwardEulerFilter  NVariant=InternalParameters  NCopyVariant=Disabled  FilterICVariant=InternalICsFilter  IntegratorICVariant=InternalICs  ExternalResetVariant=Disabled  TRSumVariant=Passthrough  SumFdbkVariant=Disabled  SumVariant=Sum_PID  TsampFilterVariant=InternalTs  TsampNgainVariant=Passthrough  TsampIntegralVariant=Passthrough  ExternalSaturationOutDataTypeStr=Inherit: Same as second input
      settings: SourceProductBaseCode=SL
  cfblk5 : Product
  cfblk6 : UnaryMinus
  cfblk7 : Sum  Inputs=+-
  cfblk8 : Gain  Gain=[902717292.421282]
  cfblk9 : Abs  SaturateOnIntegerOverflow=off
  cfblk2 : Outport
  cfblk16 : Outport  Port=2
  wires:
  cfblk14/1 -> cfblk5/1
  cfblk9/1 -> cfblk5/2
  cfblk8/1 -> cfblk9/1
  cfblk1/1 -> cfblk8/1
  cfblk13/1 -> cfblk4/1, cfblk7/2
  cfblk4/1 -> cfblk16/1
  cfblk6/1 -> cfblk10/1
  cfblk10/1 -> cfblk7/1
  cfblk3/1 -> cfblk11/1
  cfblk12/1 -> cfblk3/1
  cfblk15/1 -> cfblk6/1
  cfblk5/1 -> cfblk4/2
  cfblk7/1 -> cfblk2/1
  cfblk11/1 -> cfblk17/1
  cfblk17/1 -> cfblk3/2

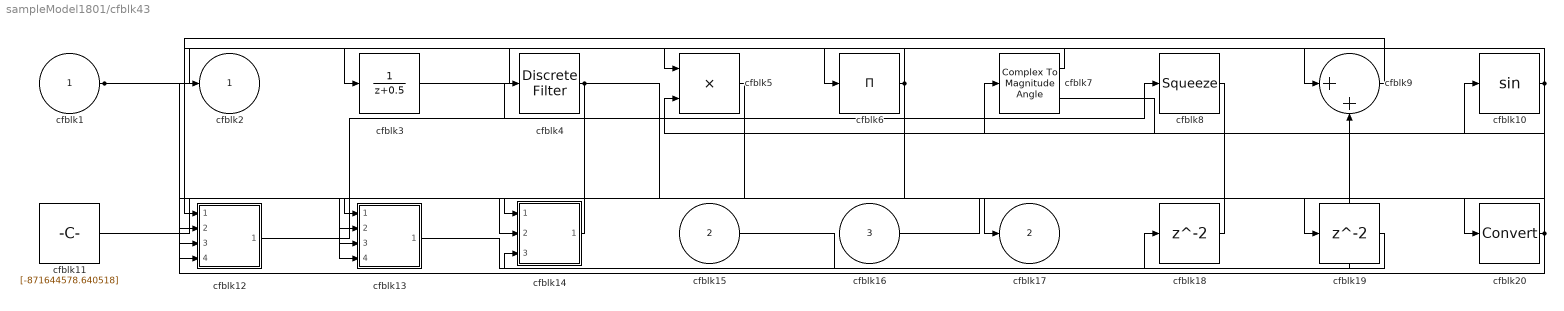
== system sampleModel1801/cfblk43 ==
  cfblk1 : Inport
  cfblk15 : Inport  Port=2
  cfblk16 : Inport  Port=3
  cfblk10 : Trigonometry
  cfblk11 : Constant  Value=[-871644578.640518]  SampleTime=1
  cfblk12 : Subsystem
  cfblk13 : Subsystem
  cfblk14 : Subsystem
  cfblk18 : Delay  SampleTime=1
  cfblk19 : Delay  SampleTime=1
  cfblk20 : DataTypeConversion  SaturateOnIntegerOverflow=off  RndMeth=Floor
  cfblk3 : DiscreteTransferFcn  SampleTime=1
  cfblk4 : DiscreteFilter  SampleTime=1
  cfblk5 : Product  Inputs=**
  cfblk6 : Product  Inputs=*
  cfblk7 : ComplexToMagnitudeAngle
  cfblk8 : Squeeze
  cfblk9 : Sum  Inputs=|++
  cfblk2 : Outport
  cfblk17 : Outport  Port=2
  wires:
  cfblk11/1 -> cfblk17/1
  cfblk16/1 -> cfblk20/1
  cfblk3/1 -> cfblk9/1
  cfblk7/1 -> cfblk6/1
  cfblk15/1 -> cfblk9/2
  cfblk9/1 -> cfblk12/1(cfblk1)
  cfblk1/1 -> cfblk3/1, cfblk13/2(cfblk7)
  cfblk12/1(cfblk2) -> cfblk8/1
  cfblk6/1 -> cfblk2/1, cfblk12/4(cfblk17), cfblk13/4(cfblk9)
  cfblk4/1 -> cfblk13/1(cfblk1), cfblk19/1
  cfblk8/1 -> cfblk14/1(cfblk1)
  cfblk5/1 -> cfblk14/2(cfblk11)
  cfblk14/1(cfblk2) -> cfblk4/1
  cfblk7/2 -> cfblk10/1
  cfblk10/1 -> cfblk5/1, cfblk5/2, cfblk13/3(cfblk8)
  cfblk13/1(cfblk2) -> cfblk18/1
  cfblk18/1 -> cfblk12/2(cfblk15)
  cfblk19/1 -> cfblk14/3(cfblk12)
  cfblk20/1 -> cfblk12/3(cfblk16), cfblk7/1

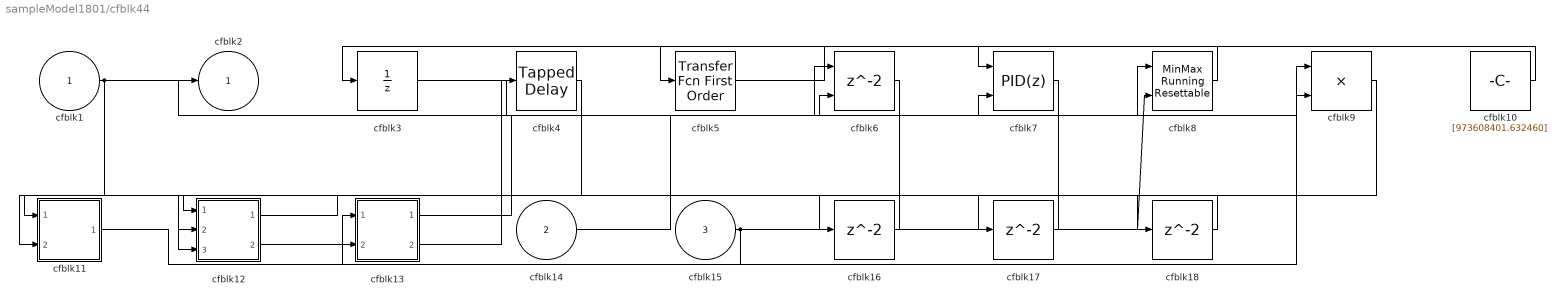
== system sampleModel1801/cfblk44 ==
  cfblk1 : Inport
  cfblk14 : Inport  Port=2
  cfblk15 : Inport  Port=3
  cfblk10 : Constant  Value=[973608401.632460]  SampleTime=1
  cfblk11 : Subsystem
  cfblk12 : Subsystem
  cfblk13 : Subsystem
  cfblk16 : Delay  SampleTime=1
  cfblk17 : Delay  SampleTime=1
  cfblk18 : Delay  SampleTime=1
  cfblk3 : UnitDelay  HasFrameUpgradeWarning=on
  cfblk4 : simulink/Discrete/Tapped Delay  vinit=0.0  samptime=-1  NumDelays=1  DelayOrder=Oldest  includeCurrent=off
  cfblk5 : simulink/Discrete/Transfer Fcn First Order  PoleZ=0.95  ICPrevOutput=0.0  DoSatur=off
  cfblk6 : Delay  ShowEnablePort=on  SampleTime=1
      settings: InputPortMap=u0,e6
  cfblk7 : slpidlib/PID Controller (2DOF)  Controller=PID  Form=Parallel  TimeDomain=Discrete-time  UseExternalTs=off  SampleTime=1  IntegratorMethod=Forward Euler  FilterMethod=Forward Euler  ControllerParametersSource=internal  P=1  I=1  UseKiTs=off  D=0  N=100  UseFilter=on  b=1  c=1  TunerSelectOption=Transfer Function Based (PID Tuner App)  InitialConditionSource=internal  InitialConditionForIntegrator=0  InitialConditionForFilter=0  DifferentiatorICPrevScaledInput=0  ExternalReset=none  TrackingMode=off  Kt=1  LimitOutput=off  SatLimitsSource=internal  UpperSaturationLimit=inf  LowerSaturationLimit=-inf  LinearizeAsGain=off  AntiWindupMode=none  Kb=1  POutMin=[]  POutMax=[]  IOutMin=[]  IOutMax=[]  DOutMin=[]  DOutMax=[]  NOutMin=[]  NOutMax=[]  bOutMin=[]  bOutMax=[]  cOutMin=[]  cOutMax=[]  SumOutMin=[]  SumOutMax=[]  SaturationOutMin=[]  SaturationOutMax=[]  PParamMin=[]  PParamMax=[]  IParamMin=[]  IParamMax=[]  DParamMin=[]  DParamMax=[]  NParamMin=[]  NParamMax=[]  bParamMin=[]  bParamMax=[]  cParamMin=[]  cParamMax=[]  KbParamMin=[]  KbParamMax=[]  KtParamMin=[]  KtParamMax=[]  KbOutMin=[]  KbOutMax=[]  KtOutMin=[]  KtOutMax=[]  IntegratorOutMin=[]  IntegratorOutMax=[]  FilterOutMin=[]  FilterOutMax=[]  SumI1OutMin=[]  SumI1OutMax=[]  SumI2OutMin=[]  SumI2OutMax=[]  SumI3OutMin=[]  SumI3OutMax=[]  SumI4OutMin=[]  SumI4OutMax=[]  SumDOutMin=[]  SumDOutMax=[]  Sum1OutMin=[]  Sum1OutMax=[]  Sum2OutMin=[]  Sum2OutMax=[]  Sum3OutMin=[]  Sum3OutMax=[]  DifferentiatorOutMin=[]  DifferentiatorOutMax=[]  FilterDiffOutCoefMin=[]  FilterDiffOutCoefMax=[]  ReciprocalOutMin=[]  ReciprocalOutMax=[]  SumDenOutMin=[]  SumDenOutMax=[]  SumNumOutMin=[]  SumNumOutMax=[]  DivideOutMin=[]  DivideOutMax=[]  UdiffTsProdOutMin=[]  UdiffTsProdOutMax=[]  NTsProdOutMin=[]  NTsProdOutMax=[]  UintegralTsProdOutMin=[]  UintegralTsProdOutMax=[]  UngainTsProdOutMin=[]  UngainTsProdOutMax=[]  IntegratorContinuousStateAttributes=''  IntegratorStateMustResolveToSignalObject=off  IntegratorRTWStateStorageClass=Auto  FilterContinuousStateAttributes=''  FilterStateMustResolveToSignalObject=off  FilterRTWStateStorageClass=Auto  ParallelPVariant=InternalParameters  IdealPVariant=Disabled  IVariant=InternalParameters  DVariant=InternalParameters  bVariant=InternalParameters  cVariant=InternalParameters  IntegratorVariant=Discrete  SatVariant=Disabled  AWVariant=Passthrough  PCopyVariant=Disabled  TRVariant=Disabled  FdbkBlocksVariant=Forward  IdealPFdbkVariant=Disabled  SatFdbkVariant=Disabled  DerivativeFilterVariant=ForwardEulerFilter  NVariant=InternalParameters  NCopyVariant=Disabled  FilterICVariant=InternalICsFilter  IntegratorICVariant=InternalICs  ExternalResetVariant=Disabled  TRSumVariant=Passthrough  SumFdbkVariant=Disabled  SumVariant=Sum_PID  TsampFilterVariant=InternalTs  TsampNgainVariant=Passthrough  TsampIntegralVariant=Passthrough  ExternalSaturationOutDataTypeStr=Inherit: Same as second input
      settings: SourceProductBaseCode=SL
  cfblk8 : simulink/Math Operations/MinMax Running Resettable  Function=min  vinit=0.0
  cfblk9 : Product
  cfblk2 : Outport
  wires:
  cfblk13/1(cfblk2) -> cfblk8/1
  cfblk5/1 -> cfblk7/1
  cfblk15/1 -> cfblk8/2, cfblk13/2(cfblk13)
  cfblk11/1(cfblk2) -> cfblk9/1
  cfblk14/1 -> cfblk7/2
  cfblk3/1 -> cfblk9/2
  cfblk8/1 -> cfblk5/1
  cfblk6/1 -> cfblk12/3(cfblk11)
  cfblk12/2(cfblk12) -> cfblk13/1(cfblk1)
  cfblk1/1 -> cfblk2/1, cfblk6/2, cfblk11/2(cfblk11)
  cfblk13/2(cfblk14) -> cfblk4/1
  cfblk10/1 -> cfblk3/1
  cfblk4/1 -> cfblk11/1(cfblk1)
  cfblk12/1(cfblk2) -> cfblk16/1
  cfblk16/1 -> cfblk6/1
  cfblk7/1 -> cfblk17/1
  cfblk17/1 -> cfblk12/2(cfblk10)
  cfblk9/1 -> cfblk18/1
  cfblk18/1 -> cfblk12/1(cfblk1)

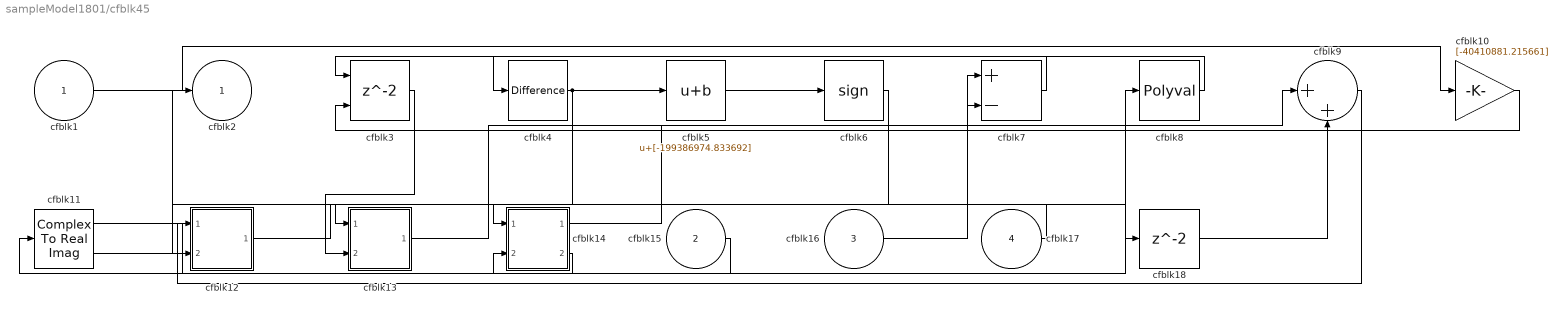
== system sampleModel1801/cfblk45 ==
  cfblk1 : Inport
  cfblk15 : Inport  Port=2
  cfblk16 : Inport  Port=3
  cfblk17 : Inport  Port=4
  cfblk10 : Gain  Gain=[-40410881.215661]
  cfblk11 : ComplexToRealImag
  cfblk12 : Subsystem
  cfblk13 : Subsystem
  cfblk14 : Subsystem
  cfblk18 : Delay  SampleTime=1
  cfblk3 : Delay  ShowEnablePort=on  SampleTime=1
      settings: InputPortMap=u0,e6
  cfblk4 : simulink/Discrete/Difference  ICPrevInput=0.0  OutMin=[]  OutMax=[]  OutDataTypeStr=Inherit: Inherit via back propagation  OutDataType=fixdt(1, 16)  OutScaling=2^-10  DoSatur=off
  cfblk5 : Bias  Bias=[-199386974.833692]  SaturateOnIntegerOverflow=off
  cfblk6 : Signum
  cfblk7 : Sum  Inputs=+-
  cfblk8 : Polyval  Coefs=[ +2.081618890e-019, -1.441693666e-014, +4.719686976e-010, -8.536869453e-006, +1.621573104e-001, -8.087801117e+001 ]
  cfblk9 : Sum  Inputs=|++
  cfblk2 : Outport
  wires:
  cfblk4/1 -> cfblk13/1(cfblk1), cfblk5/1
  cfblk8/1 -> cfblk4/1
  cfblk11/1 -> cfblk8/1
  cfblk1/1 -> cfblk10/1
  cfblk7/1 -> cfblk3/1
  cfblk3/1 -> cfblk13/2(cfblk12)
  cfblk17/1 -> cfblk14/1(cfblk1)
  cfblk9/1 -> cfblk12/1(cfblk1)
  cfblk11/2 -> cfblk2/1
  cfblk13/1(cfblk2) -> cfblk9/1
  cfblk10/1 -> cfblk3/2
  cfblk15/1 -> cfblk14/2(cfblk11)
  cfblk6/1 -> cfblk12/2(cfblk16)
  cfblk14/1(cfblk2) -> cfblk7/1
  cfblk16/1 -> cfblk7/2
  cfblk14/2(cfblk12) -> cfblk11/1
  cfblk5/1 -> cfblk6/1
  cfblk12/1(cfblk2) -> cfblk18/1
  cfblk18/1 -> cfblk9/2

== system sampleModel1801/cfblk46 ==
  cfblk1 : Inport
  cfblk11 : Inport  Port=2
  cfblk12 : Inport  Port=3
  cfblk10 : Subsystem
  cfblk3 : DiscreteFir  SampleTime=1
  cfblk4 : Delay  ShowEnablePort=on  SampleTime=1
      settings: InputPortMap=u0,e6
  cfblk5 : simulink/Math Operations/MinMax Running Resettable  Function=min  vinit=0.0
  cfblk6 : simulink/Math Operations/MinMax Running Resettable  Function=min  vinit=0.0
  cfblk7 : Sqrt  Operator=rSqrt  AlgorithmType=Newton-Raphson
  cfblk8 : Sum
  cfblk9 : Constant  Value=[908886909.241913]  SampleTime=1
  cfblk2 : Outport
  cfblk13 : Outport  Port=2
  wires:
  cfblk12/1 -> cfblk3/1
  cfblk11/1 -> cfblk5/1
  cfblk9/1 -> cfblk6/1
  cfblk8/1 -> cfblk5/2
  cfblk4/1 -> cfblk7/1
  cfblk1/1 -> cfblk10/1(cfblk1)
  cfblk3/1 -> cfblk4/1, cfblk8/2
  cfblk5/1 -> cfblk2/1
  cfblk7/1 -> cfblk6/2
  cfblk10/1(cfblk2) -> cfblk4/2
  cfblk10/2(cfblk9) -> cfblk13/1
  cfblk6/1 -> cfblk8/1

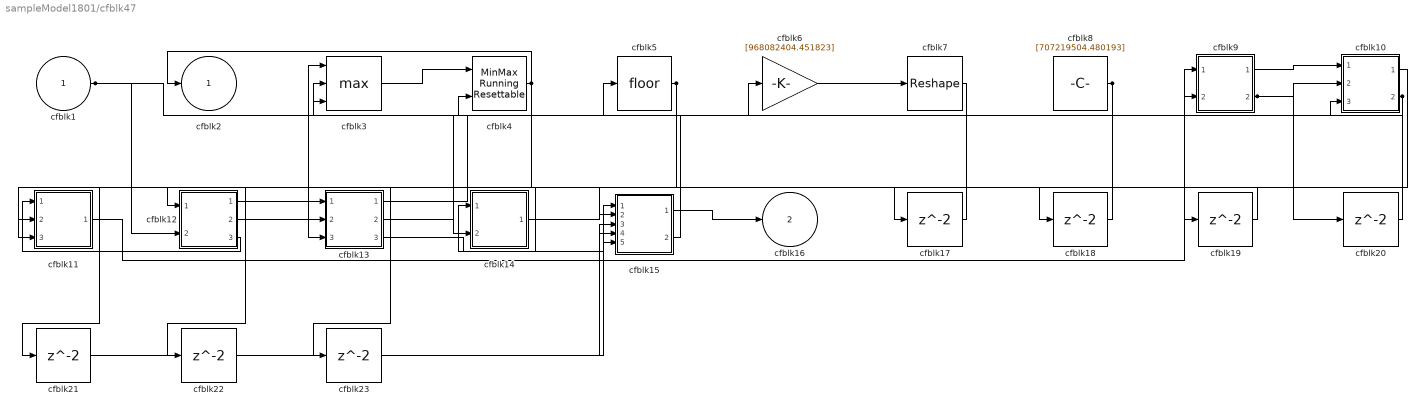
== system sampleModel1801/cfblk47 ==
  cfblk1 : Inport
  cfblk10 : Subsystem
  cfblk11 : Subsystem
  cfblk12 : Subsystem
  cfblk13 : Subsystem
  cfblk14 : Subsystem
  cfblk15 : Subsystem
  cfblk{17..23} (7 alike) : Delay  SampleTime=1
  cfblk3 : MinMax  Function=max  Inputs=3
  cfblk4 : simulink/Math Operations/MinMax Running Resettable  Function=min  vinit=0.0
  cfblk5 : Rounding
  cfblk6 : Gain  Gain=[968082404.451823]
  cfblk7 : Reshape
  cfblk8 : Constant  Value=[707219504.480193]  SampleTime=1
  cfblk9 : Subsystem
  cfblk2 : Outport
  cfblk16 : Outport  Port=2
  wires:
  cfblk13/1(cfblk2) -> cfblk6/1
  cfblk6/1 -> cfblk7/1
  cfblk8/1 -> cfblk14/1(cfblk1), cfblk13/3(cfblk10)
  cfblk4/1 -> cfblk2/1, cfblk11/2(cfblk14), cfblk21/1, cfblk22/1, cfblk23/1
  cfblk1/1 -> cfblk12/2(cfblk13), cfblk10/3(cfblk14)
  cfblk15/1(cfblk2) -> cfblk16/1
  cfblk11/1(cfblk2) -> cfblk9/1(cfblk1)
  cfblk13/2(cfblk11) -> cfblk5/1
  cfblk10/2(cfblk15) -> cfblk14/2(cfblk10), cfblk18/1
  cfblk3/1 -> cfblk4/1
  cfblk12/1(cfblk2) -> cfblk13/1(cfblk1)
  cfblk9/1(cfblk2) -> cfblk10/1(cfblk1)
  cfblk13/3(cfblk12) -> cfblk15/1(cfblk1)
  cfblk7/1 -> cfblk15/2(cfblk9)
  cfblk15/2(cfblk13) -> cfblk3/2
  cfblk5/1 -> cfblk3/3, cfblk11/3(cfblk15)
  cfblk12/2(cfblk14) -> cfblk9/2(cfblk13)
  cfblk9/2(cfblk14) -> cfblk10/2(cfblk13), cfblk20/1
  cfblk12/3(cfblk15) -> cfblk11/1(cfblk1)
  cfblk10/1(cfblk2) -> cfblk17/1
  cfblk17/1 -> cfblk12/1(cfblk1)
  cfblk18/1 -> cfblk3/1
  cfblk14/1(cfblk2) -> cfblk19/1
  cfblk19/1 -> cfblk13/2(cfblk9)
  cfblk20/1 -> cfblk4/2
  cfblk21/1 -> cfblk15/3(cfblk10)
  cfblk22/1 -> cfblk15/4(cfblk11)
  cfblk23/1 -> cfblk15/5(cfblk12)

== system sampleModel1801/cfblk48 ==
  cfblk1 : Inport
  cfblk10 : Subsystem
  cfblk11 : Subsystem
  cfblk12 : Delay  SampleTime=1
  cfblk13 : Delay  SampleTime=1
  cfblk14 : Delay  SampleTime=1
  cfblk3 : DiscreteTransferFcn  SampleTime=1
  cfblk4 : Delay  ShowEnablePort=on  SampleTime=1
      settings: InputPortMap=u0,e6
  cfblk5 : simulink/Discrete/Difference  ICPrevInput=0.0  OutMin=[]  OutMax=[]  OutDataTypeStr=Inherit: Inherit via back propagation  OutDataType=fixdt(1, 16)  OutScaling=2^-10  DoSatur=off
  cfblk6 : Squeeze
  cfblk7 : Sum  Inputs=-+
  cfblk8 : Constant  Value=[107991499.195847]  SampleTime=1
  cfblk9 : Constant  Value=[364152965.924011]  SampleTime=1
  cfblk2 : Outport
  wires:
  cfblk11/1(cfblk2) -> cfblk10/1(cfblk1)
  cfblk8/1 -> cfblk6/1
  cfblk1/1 -> cfblk11/1(cfblk1)
  cfblk9/1 -> cfblk5/1
  cfblk10/1(cfblk2) -> cfblk4/1
  cfblk5/1 -> cfblk4/2
  cfblk6/1 -> cfblk7/1
  cfblk4/1 -> cfblk3/1, cfblk12/1
  cfblk10/2(cfblk10) -> cfblk7/2, cfblk2/1
  cfblk12/1 -> cfblk11/3(cfblk12)
  cfblk3/1 -> cfblk13/1
  cfblk13/1 -> cfblk10/2(cfblk9)
  cfblk7/1 -> cfblk14/1
  cfblk14/1 -> cfblk11/2(cfblk11)

== system sampleModel1801/cfblk50 ==
  cfblk1 : Inport
  cfblk8 : Inport  Port=2
  cfblk9 : Inport  Port=3
  Action Port : ActionPort  ActionPortLabel=if(u1 >= 0)
  cfblk11 : Subsystem  TreatAsAtomicUnit=on
  cfblk12 : Subsystem  TreatAsAtomicUnit=on
  cfblk13 : Delay
  cfblk14 : Delay
  cfblk15 : Delay
  cfblk3 : simulink/Discrete/Tapped Delay  vinit=0.0  samptime=-1  NumDelays=1  DelayOrder=Oldest  includeCurrent=off
  cfblk4 : Sum  Inputs=+-
  cfblk5 : Sum  Inputs=+
  cfblk6 : Subsystem
  cfblk7 : If  IfExpression=u1 >= 0  SampleTime=1
  cfblk2 : Outport
  cfblk10 : Outport  Port=2
  wires:
  cfblk8/1 -> cfblk11/1(cfblk1), cfblk6/2(cfblk8)
  cfblk5/1 -> cfblk3/1, cfblk15/1
  cfblk6/1(cfblk2) -> cfblk4/1, cfblk5/1
  cfblk9/1 -> cfblk6/1(cfblk1)
  cfblk12/1(cfblk2) -> cfblk10/1, cfblk6/3(cfblk9), cfblk13/1
  cfblk11/1(cfblk2) -> cfblk2/1
  cfblk1/1 -> cfblk12/3(cfblk8)
  cfblk3/1 -> cfblk4/2
  cfblk7/1 -> cfblk11/Action
  cfblk7/2 -> cfblk12/Action
  cfblk13/1 -> cfblk7/1
  cfblk4/1 -> cfblk14/1
  cfblk14/1 -> cfblk12/2(cfblk7)
  cfblk15/1 -> cfblk12/1(cfblk1)

== system sampleModel1801/cfblk51 ==
  cfblk1 : Inport
  cfblk6 : Inport  Port=2
  Action Port : ActionPort  ActionPortLabel=else
  cfblk3 : Constant  Value=[-414644747.461985]  SampleTime=1
  cfblk4 : Constant  Value=[180233872.112493]  SampleTime=1
  cfblk5 : Subsystem
  cfblk2 : Outport
  cfblk7 : Outport  Port=2
  wires:
  cfblk4/1 -> cfblk7/1, cfblk5/3(cfblk12), cfblk5/4(cfblk13)
  cfblk1/1 -> cfblk5/1(cfblk1)
  cfblk6/1 -> cfblk5/2(cfblk11)
  cfblk3/1 -> cfblk2/1

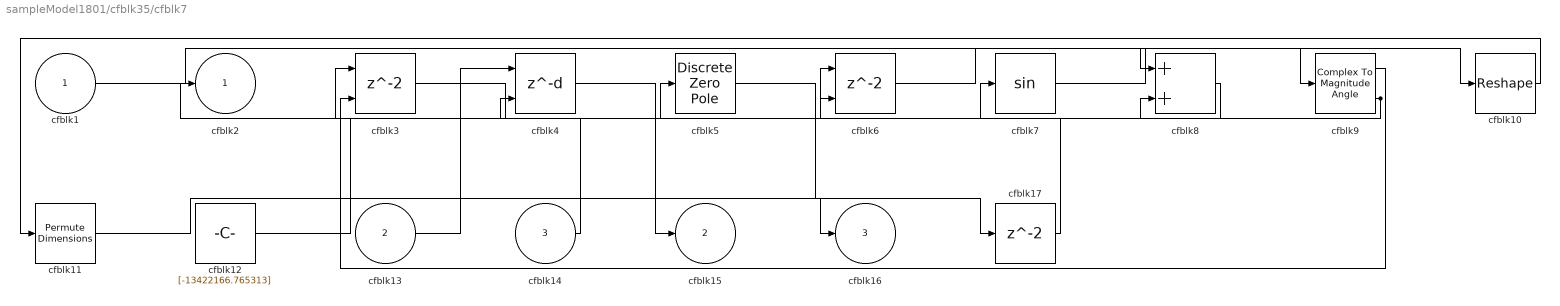
== system sampleModel1801/cfblk35/cfblk7 ==
  cfblk1 : Inport
  cfblk13 : Inport  Port=2
  cfblk14 : Inport  Port=3
  cfblk10 : Reshape
  cfblk11 : PermuteDimensions
  cfblk12 : Constant  Value=[-13422166.765313]  SampleTime=1
  cfblk17 : Delay  SampleTime=1
  cfblk3 : Delay  ShowEnablePort=on  SampleTime=1
      settings: InputPortMap=u0,e6
  cfblk4 : Delay  DelayLengthSource=Input port  SampleTime=1
      settings: InputPortMap=u0,p1
  cfblk5 : DiscreteZeroPole  Poles=[0 0.5]  Gain=1
  cfblk6 : Delay  ShowEnablePort=on  SampleTime=1
      settings: InputPortMap=u0,e6
  cfblk7 : Trigonometry
  cfblk8 : Sum
  cfblk9 : ComplexToMagnitudeAngle
  cfblk2 : Outport
  cfblk15 : Outport  Port=2
  cfblk16 : Outport  Port=3
  wires:
  cfblk1/1 -> cfblk10/1
  cfblk13/1 -> cfblk4/1
  cfblk9/1 -> cfblk3/2
  cfblk3/1 -> cfblk5/1
  cfblk12/1 -> cfblk7/1
  cfblk8/1 -> cfblk4/2
  cfblk10/1 -> cfblk11/1
  cfblk7/1 -> cfblk9/1
  cfblk4/1 -> cfblk15/1
  cfblk6/1 -> cfblk8/1
  cfblk14/1 -> cfblk2/1
  cfblk9/2 -> cfblk6/1, cfblk6/2, cfblk8/2
  cfblk11/1 -> cfblk16/1
  cfblk5/1 -> cfblk17/1
  cfblk17/1 -> cfblk3/1

== system sampleModel1801/cfblk36/cfblk10 ==
  cfblk1 : Inport
  cfblk11 : Inport  Port=2
  cfblk12 : Inport  Port=3
  cfblk10 : Constant  Value=[-885848148.818032]  SampleTime=1
  cfblk3 : simulink/Discrete/Tapped Delay  vinit=0.0  samptime=-1  NumDelays=1  DelayOrder=Oldest  includeCurrent=off
  cfblk4 : Sin  TimeSource=Use external signal  SampleTime=0
  cfblk5 : Rounding
  cfblk6 : Sum  Inputs=|++
  cfblk7 : simulink/Math Operations/MinMax Running Resettable  Function=min  vinit=0.0
  cfblk8 : Sqrt  Operator=rSqrt  AlgorithmType=Newton-Raphson
  cfblk9 : Abs  SaturateOnIntegerOverflow=off
  cfblk2 : Outport
  wires:
  cfblk11/1 -> cfblk5/1
  cfblk3/1 -> cfblk2/1
  cfblk8/1 -> cfblk9/1
  cfblk10/1 -> cfblk8/1
  cfblk9/1 -> cfblk6/1
  cfblk12/1 -> cfblk6/2
  cfblk1/1 -> cfblk7/1
  cfblk7/1 -> cfblk3/1
  cfblk6/1 -> cfblk4/1
  cfblk5/1 -> cfblk7/2

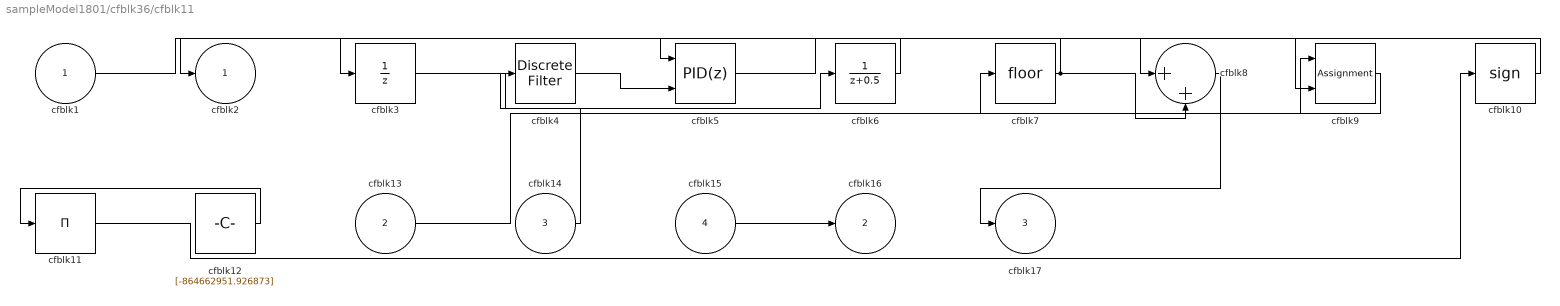
== system sampleModel1801/cfblk36/cfblk11 ==
  cfblk1 : Inport
  cfblk13 : Inport  Port=2
  cfblk14 : Inport  Port=3
  cfblk15 : Inport  Port=4
  cfblk10 : Signum
  cfblk11 : Product  Inputs=*
  cfblk12 : Constant  Value=[-864662951.926873]  SampleTime=1
  cfblk3 : UnitDelay  HasFrameUpgradeWarning=on
  cfblk4 : DiscreteFilter  SampleTime=1
  cfblk5 : slpidlib/PID Controller (2DOF)  Controller=PID  Form=Parallel  TimeDomain=Discrete-time  UseExternalTs=off  SampleTime=1  IntegratorMethod=Forward Euler  FilterMethod=Forward Euler  ControllerParametersSource=internal  P=1  I=1  UseKiTs=off  D=0  N=100  UseFilter=on  b=1  c=1  TunerSelectOption=Transfer Function Based (PID Tuner App)  InitialConditionSource=internal  InitialConditionForIntegrator=0  InitialConditionForFilter=0  DifferentiatorICPrevScaledInput=0  ExternalReset=none  TrackingMode=off  Kt=1  LimitOutput=off  SatLimitsSource=internal  UpperSaturationLimit=inf  LowerSaturationLimit=-inf  LinearizeAsGain=off  AntiWindupMode=none  Kb=1  POutMin=[]  POutMax=[]  IOutMin=[]  IOutMax=[]  DOutMin=[]  DOutMax=[]  NOutMin=[]  NOutMax=[]  bOutMin=[]  bOutMax=[]  cOutMin=[]  cOutMax=[]  SumOutMin=[]  SumOutMax=[]  SaturationOutMin=[]  SaturationOutMax=[]  PParamMin=[]  PParamMax=[]  IParamMin=[]  IParamMax=[]  DParamMin=[]  DParamMax=[]  NParamMin=[]  NParamMax=[]  bParamMin=[]  bParamMax=[]  cParamMin=[]  cParamMax=[]  KbParamMin=[]  KbParamMax=[]  KtParamMin=[]  KtParamMax=[]  KbOutMin=[]  KbOutMax=[]  KtOutMin=[]  KtOutMax=[]  IntegratorOutMin=[]  IntegratorOutMax=[]  FilterOutMin=[]  FilterOutMax=[]  SumI1OutMin=[]  SumI1OutMax=[]  SumI2OutMin=[]  SumI2OutMax=[]  SumI3OutMin=[]  SumI3OutMax=[]  SumI4OutMin=[]  SumI4OutMax=[]  SumDOutMin=[]  SumDOutMax=[]  Sum1OutMin=[]  Sum1OutMax=[]  Sum2OutMin=[]  Sum2OutMax=[]  Sum3OutMin=[]  Sum3OutMax=[]  DifferentiatorOutMin=[]  DifferentiatorOutMax=[]  FilterDiffOutCoefMin=[]  FilterDiffOutCoefMax=[]  ReciprocalOutMin=[]  ReciprocalOutMax=[]  SumDenOutMin=[]  SumDenOutMax=[]  SumNumOutMin=[]  SumNumOutMax=[]  DivideOutMin=[]  DivideOutMax=[]  UdiffTsProdOutMin=[]  UdiffTsProdOutMax=[]  NTsProdOutMin=[]  NTsProdOutMax=[]  UintegralTsProdOutMin=[]  UintegralTsProdOutMax=[]  UngainTsProdOutMin=[]  UngainTsProdOutMax=[]  IntegratorContinuousStateAttributes=''  IntegratorStateMustResolveToSignalObject=off  IntegratorRTWStateStorageClass=Auto  FilterContinuousStateAttributes=''  FilterStateMustResolveToSignalObject=off  FilterRTWStateStorageClass=Auto  ParallelPVariant=InternalParameters  IdealPVariant=Disabled  IVariant=InternalParameters  DVariant=InternalParameters  bVariant=InternalParameters  cVariant=InternalParameters  IntegratorVariant=Discrete  SatVariant=Disabled  AWVariant=Passthrough  PCopyVariant=Disabled  TRVariant=Disabled  FdbkBlocksVariant=Forward  IdealPFdbkVariant=Disabled  SatFdbkVariant=Disabled  DerivativeFilterVariant=ForwardEulerFilter  NVariant=InternalParameters  NCopyVariant=Disabled  FilterICVariant=InternalICsFilter  IntegratorICVariant=InternalICs  ExternalResetVariant=Disabled  TRSumVariant=Passthrough  SumFdbkVariant=Disabled  SumVariant=Sum_PID  TsampFilterVariant=InternalTs  TsampNgainVariant=Passthrough  TsampIntegralVariant=Passthrough  ExternalSaturationOutDataTypeStr=Inherit: Same as second input
      settings: SourceProductBaseCode=SL
  cfblk6 : DiscreteTransferFcn  SampleTime=1
  cfblk7 : Rounding
  cfblk8 : Sum  Inputs=|++
  cfblk9 : Assignment  DiagnosticForDimensions=Warning  IndexOptions=Index vector (dialog)  Indices=1  OutputSizes=1
  cfblk2 : Outport
  cfblk16 : Outport  Port=2
  cfblk17 : Outport  Port=3
  wires:
  cfblk10/1 -> cfblk8/1
  cfblk6/1 -> cfblk2/1
  cfblk15/1 -> cfblk16/1
  cfblk9/1 -> cfblk7/1
  cfblk3/1 -> cfblk6/1
  cfblk13/1 -> cfblk9/1
  cfblk7/1 -> cfblk8/2, cfblk3/1
  cfblk1/1 -> cfblk5/1
  cfblk14/1 -> cfblk4/1
  cfblk5/1 -> cfblk9/2
  cfblk11/1 -> cfblk10/1
  cfblk8/1 -> cfblk17/1
  cfblk4/1 -> cfblk5/2
  cfblk12/1 -> cfblk11/1

== system sampleModel1801/cfblk36/cfblk12 ==
  cfblk1 : Inport
  cfblk11 : Inport  Port=2
  cfblk12 : Inport  Port=3
  cfblk13 : Inport  Port=4
  cfblk14 : Inport  Port=5
  cfblk15 : Inport  Port=6
  cfblk10 : Abs  SaturateOnIntegerOverflow=off
  cfblk16 : Delay  SampleTime=1
  cfblk17 : Delay  SampleTime=1
  cfblk3 : UnitDelay  HasFrameUpgradeWarning=on
  cfblk4 : Delay  DelayLengthSource=Input port  SampleTime=1
      settings: InputPortMap=u0,p1
  cfblk5 : DiscreteStateSpace
  cfblk6 : simulink/Discrete/Transfer Fcn Real Zero  ZeroZ=0.75  ICPrevInput=0.0  DoSatur=off
      settings: SourceProductBaseCode=SL
  cfblk7 : Sin  TimeSource=Use external signal  SampleTime=0
  cfblk8 : simulink/Math Operations/Slider Gain  gain=1  low=0  high=2
  cfblk9 : ComplexToRealImag
  cfblk2 : Outport
  wires:
  cfblk11/1 -> cfblk5/1
  cfblk4/1 -> cfblk9/1
  cfblk14/1 -> cfblk7/1
  cfblk13/1 -> cfblk6/1
  cfblk8/1 -> cfblk10/1
  cfblk5/1 -> cfblk2/1
  cfblk1/1 -> cfblk3/1
  cfblk7/1 -> cfblk4/2
  cfblk9/1 -> cfblk16/1
  cfblk16/1 -> cfblk4/1
  cfblk10/1 -> cfblk17/1
  cfblk17/1 -> cfblk8/1

== system sampleModel1801/cfblk36/cfblk13 ==
  cfblk1 : Inport
  cfblk8 : Inport  Port=2
  cfblk11 : Delay  SampleTime=1
  cfblk3 : Gain  Gain=[-374366867.559972]
  cfblk4 : Polyval  Coefs=[ +2.081618890e-019, -1.441693666e-014, +4.719686976e-010, -8.536869453e-006, +1.621573104e-001, -8.087801117e+001 ]
  cfblk5 : DotProduct  OutDataTypeStr=Inherit: Inherit via internal rule
  cfblk6 : ComplexToRealImag
  cfblk7 : Constant  Value=[-361928093.125990]  SampleTime=1
  cfblk2 : Outport
  cfblk9 : Outport  Port=2
  cfblk10 : Outport  Port=3
  wires:
  cfblk7/1 -> cfblk5/1
  cfblk1/1 -> cfblk10/1
  cfblk3/1 -> cfblk2/1
  cfblk8/1 -> cfblk6/1
  cfblk4/1 -> cfblk5/2
  cfblk6/1 -> cfblk3/1
  cfblk6/2 -> cfblk9/1
  cfblk5/1 -> cfblk11/1
  cfblk11/1 -> cfblk4/1

== system sampleModel1801/cfblk38/cfblk10 ==
  cfblk1 : Inport
  cfblk11 : Inport  Port=2
  cfblk10 : Constant  Value=[-434416693.536615]  SampleTime=1
  cfblk3 : Delay  SampleTime=1
  cfblk4 : DiscreteStateSpace
  cfblk5 : DiscreteZeroPole  Poles=[0 0.5]  Gain=1
  cfblk6 : ComplexToMagnitudeAngle
  cfblk7 : MinMax  Function=max  Inputs=2
  cfblk8 : simulink/Math Operations/Slider Gain  gain=1  low=0  high=2
  cfblk9 : Constant  Value=[265791829.871005]  SampleTime=1
  cfblk2 : Outport
  wires:
  cfblk6/1 -> cfblk3/1
  cfblk9/1 -> cfblk8/1
  cfblk7/1 -> cfblk4/1
  cfblk3/1 -> cfblk7/1
  cfblk5/1 -> cfblk6/1
  cfblk11/1 -> cfblk5/1
  cfblk1/1 -> cfblk2/1
  cfblk8/1 -> cfblk7/2
